simulink model "Control_Plant_Simulation_2018b"  (R2018b)
settings: Solver=VariableStepAuto  StartTime=0.0  StopTime=100  RelTol=1e-3
values from neighbouring files (symbols this model uses):
  A = [0 1 0 0;-c/th1 -(d1+d)/th1 -c/th1 -d/th1;0 0 0 1; -c/th2 -d/th2 -c/th2 -(d2+d)/th2]    [plant_control.m]
  B = [0 0;kt1/th1 0; 0 0; 0 kt2/th2]    [plant_control.m]
  C = [1 0 0 0; 0 0 1 0]    [plant_control.m]
  D = [0 0;0 0]    [plant_control.m]
undefined symbols (not defined in the file or in its folder): A1, Aobs, Bobs, Cobs, Dobs, k1, ke, kei, ki, ki2, kn, kpi, PI, PO
settings Model: Creator=Desktop  LastModifiedBy=Desktop
settings DataIOCC: ReturnWorkspaceOutputs=on
settings DebuggingCC: SFMachineParentedDataDiag=error

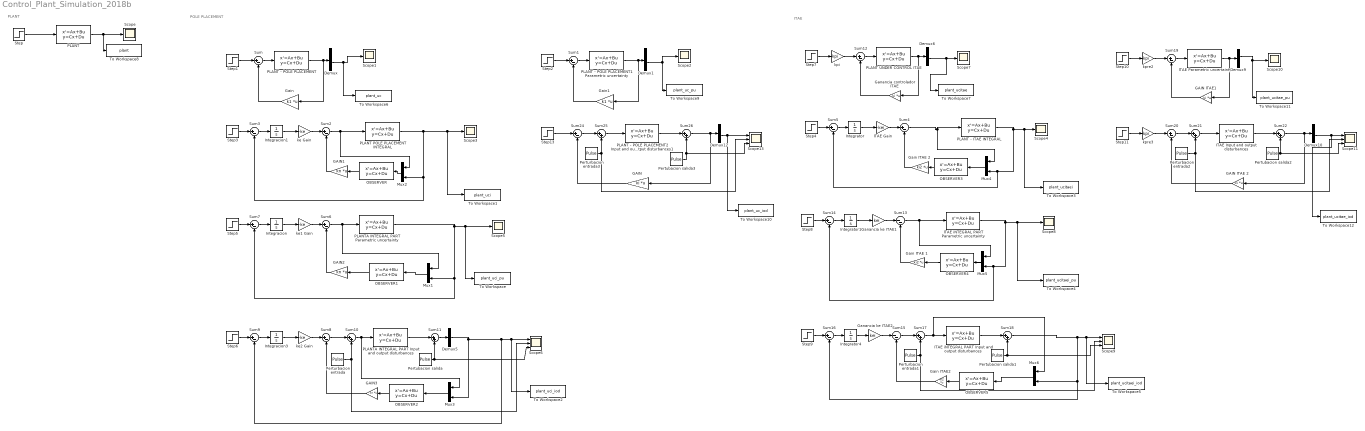
== system Control_Plant_Simulation_2018b ==
  note: PLANT
  note: ITAE
  note: POLE PLACEMENT
  " PLANT UNDER CONTROL ITAE" : StateSpace  A=A  B=B  C=eye(4)  D=[0;0;0;0]  InitialCondition=0
  Demux{,1,6,9..10,12} (6 alike) : Demux
  Demux5 : Demux  Outputs=1
  "GAIN " : Gain  Gain=ki  Multiplication=Matrix(K*u)
  GAIN ITAE 2 : Gain  Gain=ki  Multiplication=Matrix(K*u)
  GAIN ITAE1 : Gain  Gain=ki  Multiplication=Matrix(K*u)
  GAIN1 : Gain  Gain=kn  Multiplication=Matrix(K*u)
  GAIN2 : Gain  Gain=kn  Multiplication=Matrix(K*u)
  GAIN3 : Gain  Gain=kn  Multiplication=Matrix(K*u)
  Gain : Gain  Gain=k1  Multiplication=Matrix(K*u)
  Gain ITAE 1 : Gain  Gain=ki2  Multiplication=Matrix(K*u)
  Gain ITAE 2 : Gain  Gain=ki2  Multiplication=Matrix(K*u)
  Gain ITAE2 : Gain  Gain=ki2  Multiplication=Matrix(K*u)
  Gain1 : Gain  Gain=k1  Multiplication=Matrix(K*u)
  Ganancia controlador ITAE : Gain  Gain=ki  Multiplication=Matrix(K*u)
  Ganancia ke ITAE1 : Gain  Gain=kei
  Ganancia ke ITAE2 : Gain  Gain=kei
  ITAE Input and output disturbances : StateSpace  A=A  B=B  C=eye(4)  D=[0;0;0;0]  InitialCondition=0
  ITAE Parametric uncertainty : StateSpace  A=A1  B=B  C=eye(4)  D=[0;0;0;0]  InitialCondition=0
  ITAE Gain : Gain  Gain=-kei
  ITAE iNTEGRAL PART Input and output disturbances : StateSpace  A=A  B=B  C=C  D=D  InitialCondition=0
  ITAE iNTEGRAL PART Parametric uncertainty : StateSpace  A=A1  B=B  C=C  D=D  InitialCondition=0
  Integracion : Integrator
  Integracion1 : Integrator
  Integracion3 : Integrator
  Integrator : Integrator
  Integrator1 : Integrator
  Integrator4 : Integrator
  Mux{1..6} (6 alike) : Mux  Inputs=2
  OBSERVER{,1..5} (6 alike) : StateSpace  A=Aobs  B=Bobs  C=Cobs  D=Dobs  InitialCondition=0
  PLANT : StateSpace  A=A  B=B  C=C  D=D  InitialCondition=0
  PLANT POLE PLACEMENT INTEGRAL : StateSpace  A=A  B=B  C=C  D=D  InitialCondition=0
  PLANT - ITAE INTEGRAL : StateSpace  A=A  B=B  C=C  D=D  InitialCondition=0
  PLANT - POLE PLACEMENT : StateSpace  A=A  B=B  C=eye(4)  D=[0;0;0;0]  InitialCondition=0
  PLANT - POLE PLACEMENT1 Parametric uncertainty : StateSpace  A=A1  B=B  C=eye(4)  D=[0;0;0;0]  InitialCondition=0
  PLANT - POLE PLACEMENT2 Input and output disturbances1 : StateSpace  A=A  B=B  C=eye(4)  D=[0;0;0;0]  InitialCondition=0
  PLANTA INTEGRAL PART Input and output disturbances : StateSpace  A=A  B=B  C=C  D=D  InitialCondition=0
  PLANTA INTEGRAL PART Parametric uncertainty : StateSpace  A=A1  B=B  C=C  D=D  InitialCondition=0
  Pertubacion salida : DiscretePulseGenerator  PulseType=Time based  Amplitude=0.05  Period=20  PulseWidth=2  PhaseDelay=0.8
  Pertubacion salida1 : DiscretePulseGenerator  PulseType=Time based  Amplitude=PO  Period=20  PulseWidth=2  PhaseDelay=0.4
  Pertubacion salida2 : DiscretePulseGenerator  PulseType=Time based  Amplitude=PO  Period=20  PulseWidth=2  PhaseDelay=0.8
  Pertubacion salida3 : DiscretePulseGenerator  PulseType=Time based  Amplitude=PO  Period=20  PulseWidth=2  PhaseDelay=0.8
  Perturbacion entrada : DiscretePulseGenerator  PulseType=Time based  Amplitude=PI  Period=20  PulseWidth=2  PhaseDelay=0.3
  Perturbacion entrada1 : DiscretePulseGenerator  PulseType=Time based  Amplitude=PI  Period=20  PulseWidth=2  PhaseDelay=0.1
  Perturbacion entrada2 : DiscretePulseGenerator  PulseType=Time based  Amplitude=PI  Period=20  PulseWidth=2  PhaseDelay=0.4
  Perturbacion entrada3 : DiscretePulseGenerator  PulseType=Time based  Amplitude=PI  Period=20  PulseWidth=2  PhaseDelay=0.4
  Scope{,1..5,7..8,10} (9 alike) : Scope
  Scope{6,9,11,13} (4 alike) : Scope  NumInputPorts=3
  Step : Step  SampleTime=0
  Step{1,3..11} (10 alike) : Step  Time=0  SampleTime=0
  Step13 : Step  SampleTime=0
  Step2 : Step  SampleTime=0
  Sum{,1..9,12,14,16,19..20,24} (16 alike) : Sum  Inputs=|+-
  Sum{10..11,17..18,21..22,25..26} (8 alike) : Sum  Inputs=|++
  Sum13 : Sum  Inputs=|--
  Sum15 : Sum  Inputs=|--
  To Workspace : ToWorkspace  VariableName=plant_uci_pu  SaveFormat=Timeseries  SampleTime=-1
  To Workspace1 : ToWorkspace  VariableName=plant_uci  SaveFormat=Timeseries  SampleTime=-1
  To Workspace10 : ToWorkspace  VariableName=plant_uc_iod  SaveFormat=Timeseries  SampleTime=-1
  To Workspace11 : ToWorkspace  VariableName=plant_ucitae_pu  SaveFormat=Timeseries  SampleTime=-1
  To Workspace12 : ToWorkspace  VariableName=plant_ucitae_iod  SaveFormat=Timeseries  SampleTime=-1
  To Workspace2 : ToWorkspace  VariableName=plant_uci_iod  SaveFormat=Timeseries  SampleTime=-1
  To Workspace3 : ToWorkspace  VariableName=plant_ucitaei  SaveFormat=Timeseries  SampleTime=-1
  To Workspace4 : ToWorkspace  VariableName=plant_ucitaei_pu  SaveFormat=Timeseries  SampleTime=-1
  To Workspace5 : ToWorkspace  VariableName=plant_ucitaei_iod  SaveFormat=Timeseries  SampleTime=-1
  To Workspace6 : ToWorkspace  VariableName=plant_uc  SaveFormat=Timeseries  SampleTime=-1
  To Workspace7 : ToWorkspace  VariableName=plant_ucitae  SaveFormat=Timeseries  SampleTime=-1
  To Workspace8 : ToWorkspace  VariableName=plant  SaveFormat=Timeseries  SampleTime=-1
  To Workspace9 : ToWorkspace  VariableName=plant_uc_pu  SaveFormat=Timeseries  SampleTime=-1
  ke Gain : Gain  Gain=-ke
  ke1 Gain : Gain  Gain=-ke
  ke2 Gain : Gain  Gain=-ke
  kpi : Gain  Gain=kpi
  kpre2 : Gain  Gain=kpi
  kpre3 : Gain  Gain=kpi
  wires:
  Demux10/3 -> To Workspace12/1, Scope11/1
  Integrator4/1 -> Ganancia ke ITAE2/1
  Demux/3 -> To Workspace6/1, Scope1/1
  kpre2/1 -> Sum19/1
  Perturbacion entrada2/1 -> Scope11/2, Sum21/2
  Integrator1/1 -> Ganancia ke ITAE1/1
  Sum11/1 -> Demux5/1
  Pertubacion salida2/1 -> Scope11/3, Sum22/2
  Step11/1 -> kpre3/1
  Mux3/1 -> OBSERVER2/1
  Sum22/1 -> GAIN ITAE 2/1, Demux10/1
  Demux6/3 -> To Workspace7/1, Scope7/1
  kpre3/1 -> Sum20/1
  Sum15/1 -> Sum17/1
  GAIN ITAE 2/1 -> Sum20/2
  Step5/1 -> Sum7/1
  Sum20/1 -> Sum21/1
  Sum10/1 -> Mux3/1, PLANTA INTEGRAL PART Input and output disturbances/1
  Demux9/2 -> To Workspace11/1, Scope10/1
  Mux6/1 -> OBSERVER5/1
  Perturbacion entrada/1 -> Scope6/2, Sum10/2
  Sum21/1 -> ITAE Input and output disturbances/1
  ITAE iNTEGRAL PART Input and output disturbances/1 -> Sum18/1
  Sum16/1 -> Integrator4/1
  Sum17/1 -> Mux6/1, ITAE iNTEGRAL PART Input and output disturbances/1
  GAIN ITAE1/1 -> Sum19/2
  Pertubacion salida1/1 -> Sum18/2, Scope9/3
  Step10/1 -> kpre2/1
  Perturbacion entrada1/1 -> Scope9/2, Sum17/2
  Sum14/1 -> Integrator1/1
  Ganancia controlador ITAE/1 -> Sum12/2
  ITAE Gain/1 -> Sum4/1
  Ganancia ke ITAE2/1 -> Sum15/1
  Ganancia ke ITAE1/1 -> Sum13/1
  PLANTA INTEGRAL PART Input and output disturbances/1 -> Sum11/1
  Mux5/1 -> OBSERVER4/1
  Step8/1 -> Sum14/1
  Gain ITAE2/1 -> Sum15/2
  Step9/1 -> Sum16/1
  Sum12/1 -> " PLANT UNDER CONTROL ITAE"/1
  Sum13/1 -> Mux5/1, ITAE iNTEGRAL PART Parametric uncertainty/1
  Gain ITAE 1/1 -> Sum13/2
  PLANT POLE PLACEMENT INTEGRAL/1 -> Sum3/2, Mux2/2, To Workspace1/1, Scope3/1
  Sum/1 -> PLANT - POLE PLACEMENT/1
  kpi/1 -> Sum12/1
  " PLANT UNDER CONTROL ITAE"/1 -> Ganancia controlador ITAE/1, Demux6/1
  Sum4/1 -> Mux4/1, PLANT - ITAE INTEGRAL/1
  Sum5/1 -> Integrator/1
  Gain ITAE 2/1 -> Sum4/2
  Pertubacion salida/1 -> Sum11/2, Scope6/3
  Integrator/1 -> ITAE Gain/1
  Integracion3/1 -> ke2 Gain/1
  Sum9/1 -> Integracion3/1
  Step4/1 -> Sum5/1
  Sum6/1 -> Mux1/1, PLANTA INTEGRAL PART Parametric uncertainty/1
  Sum19/1 -> ITAE Parametric uncertainty/1
  Sum8/1 -> Sum10/1
  Mux1/1 -> OBSERVER1/1
  GAIN3/1 -> Sum8/2
  Integracion/1 -> ke1 Gain/1
  ke1 Gain/1 -> Sum6/1
  Sum7/1 -> Integracion/1
  Sum2/1 -> Mux2/1, PLANT POLE PLACEMENT INTEGRAL/1
  Demux5/1 -> Mux3/2, Sum9/2, To Workspace2/1, Scope6/1
  GAIN2/1 -> Sum6/2
  GAIN1/1 -> Sum2/2
  Step6/1 -> Sum9/1
  Step7/1 -> kpi/1
  Step1/1 -> Sum/1
  ke Gain/1 -> Sum2/1
  Gain/1 -> Sum/2
  PLANT/1 -> To Workspace8/1, Scope/1
  PLANT - POLE PLACEMENT/1 -> Gain/1, Demux/1
  ITAE Input and output disturbances/1 -> Sum22/1
  ke2 Gain/1 -> Sum8/1
  Sum3/1 -> Integracion1/1
  ITAE Parametric uncertainty/1 -> GAIN ITAE1/1, Demux9/1
  Step/1 -> PLANT/1
  Step3/1 -> Sum3/1
  PLANT - POLE PLACEMENT1 Parametric uncertainty/1 -> Gain1/1, Demux1/1
  Sum1/1 -> PLANT - POLE PLACEMENT1 Parametric uncertainty/1
  Step2/1 -> Sum1/1
  Demux1/3 -> To Workspace9/1, Scope2/1
  Gain1/1 -> Sum1/2
  Demux12/3 -> Scope13/1, To Workspace10/1
  Sum25/1 -> PLANT - POLE PLACEMENT2 Input and output disturbances1/1
  PLANT - POLE PLACEMENT2 Input and output disturbances1/1 -> Sum26/1
  Step13/1 -> Sum24/1
  Pertubacion salida3/1 -> Scope13/3, Sum26/2
  "GAIN "/1 -> Sum24/2
  Sum24/1 -> Sum25/1
  Perturbacion entrada3/1 -> Scope13/2, Sum25/2
  Sum26/1 -> "GAIN "/1, Demux12/1
  Integracion1/1 -> ke Gain/1
  OBSERVER/1 -> GAIN1/1
  Mux2/1 -> OBSERVER/1
  OBSERVER1/1 -> GAIN2/1
  PLANTA INTEGRAL PART Parametric uncertainty/1 -> Scope5/1, To Workspace/1, Mux1/2, Sum7/2
  OBSERVER2/1 -> GAIN3/1
  OBSERVER3/1 -> Gain ITAE 2/1
  Mux4/1 -> OBSERVER3/1
  PLANT - ITAE INTEGRAL/1 -> Sum5/2, Mux4/2, To Workspace3/1, Scope4/1
  ITAE iNTEGRAL PART Parametric uncertainty/1 -> Sum14/2, Mux5/2, To Workspace4/1, Scope8/1
  OBSERVER4/1 -> Gain ITAE 1/1
  Sum18/1 -> Sum16/2, Mux6/2, To Workspace5/1, Scope9/1
  OBSERVER5/1 -> Gain ITAE2/1
